simulink model "Nonlinear_Performance_Simulation_NAPE_ANTONIO_CAROTENUTO"  (R2023b)
settings: Solver=ode45  StartTime=0.0  StopTime=305.0  RelTol=1e-3  AbsTol=1e-6
undefined symbols (not defined in the file or in its folder): alpha0L, altitude_0, bankAngle_0, bankAngleMax, flightPathAngle_0, flightPathAngle_c1, flightPathAngle_c2, flightPathAngle_c3, flightPathAngle_c4, headingAngle_0, headingAngle_c1, headingAngle_c2, headingAngle_c3, headingAngle_c4, kD0, kD1, kL, kLI, kLP, kNu, kTI, kTP, kWdot, lift_0, mass_0, pL, pNu, pT, speed_0, speed_c1, speed_c2, speed_c3, speed_c4, thrust_0, thrustMax, wind_0, xE_0, yE_0
libraries: aerolibatmos2 x1
settings Model: Creator=agodemar  LastModifiedBy=sasi
settings SolverCC: AutoScaleAbsTol=off  AlgebraicLoopSolver=TrustRegion
settings DataIOCC: SaveFormat=Array  SignalLoggingSaveFormat=ModelDataLogs  ReturnWorkspaceOutputs=off
settings OptimizationCC: BlockReduction=off  BooleanDataType=off  LifeSpan=inf
settings DebuggingCC: SaveWithParameterizedLinksMsg=none  UnderspecifiedInitializationDetection=Classic  MergeDetectMultiDrivingBlocksExec=none  SignalResolutionControl=TryResolveAllWithWarning  MultiTaskDSMMsg=warning  MultiTaskCondExecSysMsg=none  UnconnectedInputMsg=warning  UnconnectedOutputMsg=warning  UnconnectedLineMsg=warning  SFUnexpectedBacktrackingDiag=warning  SFNoUnconditionalDefaultTransitionDiag=warning  ArithmeticOperatorsInVariantConditions=warning
settings HardwareCC: TargetUnknown=on
settings ModelReferenceCC: EnableRefExpFcnMdlSchedulingChecks=on  PropagateSignalLabelsOutOfModel=off
settings SFSimCC: SimUseLocalCustomCode=off  CustomCodeUndefinedFunction=UseInterfaceOnly
settings RTWCC: RTWUseLocalCustomCode=off
settings CodeAppCC: StateflowObjectComments=on
settings GRTTargetCC: TargetLangStandard=C89/C90 (ANSI)  CombineOutputUpdateFcns=off  GRTInterface=on
settings ConfigComp: CovMetricSettings=dw  CovSaveCumulativeToWorkspaceVar=on  CovSaveSingleToWorkspaceVar=on  CovExternalEMLEnable=off

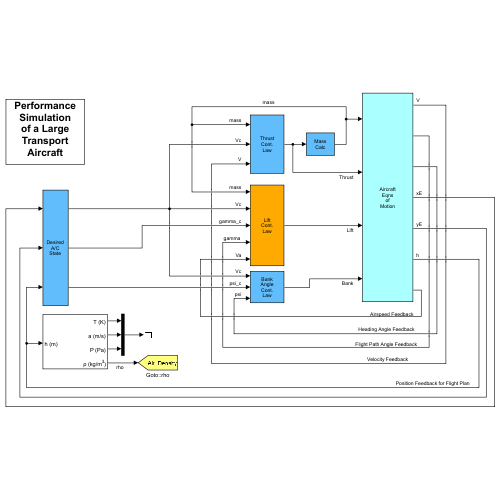
[thumbnail: Simulink's stored preview of the top-level diagram]
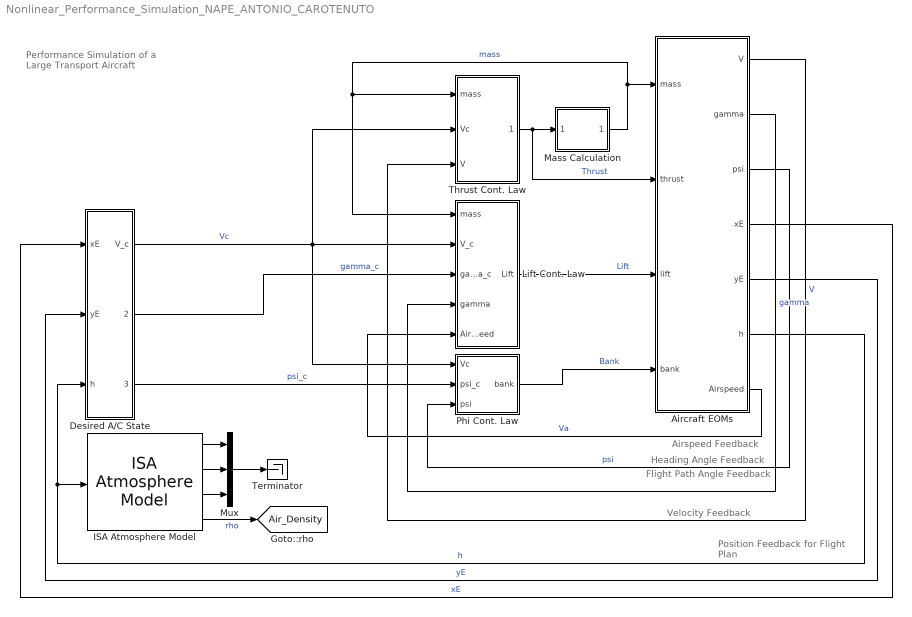
== system Nonlinear_Performance_Simulation_NAPE_ANTONIO_CAROTENUTO ==
  note: Performance Simulation
      | of a Large Transport Aircraft
  note: Velocity Feedback
  note: Flight Path Angle Feedback
  note: Heading Angle Feedback
  note: Position Feedback for Flight Plan
  note: Airspeed Feedback
  Aircraft EOMs : Subsystem
      mask Display: disp('Aircraft\nEqns\nof\nMotion')
  Desired A/C State : Subsystem
      mask Display: disp('Desired\nA/C\nState')
  ISA Atmosphere Model : aerolibatmos2/ISA Atmosphere Model  useExtended=off  action=Warning  custom=off  viscosityOut=off  g=9.80665  gamma=1.4  R=287.0531  L=0.0065  h_trop=11000  h_strat=20000  rho0=1.225  P0=101325  T0=288.15  h0=0
  Lift Cont. Law : Subsystem
      mask Display: disp('Lift\nCont.\nLaw')
  Mass Calculation : Subsystem
      mask Display: disp('Mass\nCalc')
  Mux : Mux  Inputs=3
  Phi Cont. Law : Subsystem
      mask Display: disp('Bank\nAngle\nCont.\nLaw')
  Terminator : Terminator
  Thrust Cont. Law : Subsystem
      mask Display: disp('Thrust\nCont.\nLaw')
  tag scope: Air_Density=global
  wires:
  Phi Cont. Law/1(bank) -> Aircraft EOMs/4(bank)  "Bank"
  Mass Calculation/1("Mass ") -> Lift Cont. Law/1(mass), Thrust Cont. Law/1(mass), Aircraft EOMs/1("mass ")  "mass"
  Lift Cont. Law/1(Lift) -> Aircraft EOMs/3("lift ")  "Lift"
  Thrust Cont. Law/1(Thrust) -> Aircraft EOMs/2("thrust "), Mass Calculation/1(thrust)  "Thrust"
  Desired A/C State/1(V_c) -> Phi Cont. Law/1(Vc), Thrust Cont. Law/2(Vc), Lift Cont. Law/2(V_c)  "Vc"
  Desired A/C State/2(gamma_c) -> Lift Cont. Law/3(gamma_c)  "gamma_c"
  Desired A/C State/3(psi_c) -> Phi Cont. Law/2(psi_c)  "psi_c"
  Aircraft EOMs/3(" psi ") -> Phi Cont. Law/3(psi)  "psi"
  Aircraft EOMs/2(" gamma ") -> Lift Cont. Law/4(gamma)  "gamma"
  Aircraft EOMs/1(" V ") -> Thrust Cont. Law/3(V)  "V"
  Aircraft EOMs/7(Airspeed) -> Lift Cont. Law/5(Airspeed)  "Va"
  Aircraft EOMs/6(h) -> Desired A/C State/3(h), ISA Atmosphere Model/1  "h"
  Aircraft EOMs/5(yE) -> Desired A/C State/2(yE)  "yE"
  Aircraft EOMs/4(xE) -> Desired A/C State/1(xE)  "xE"
  Mux/1 -> Terminator/1
  ISA Atmosphere Model/1 -> Mux/1
  ISA Atmosphere Model/2 -> Mux/2
  ISA Atmosphere Model/3 -> Mux/3
  ISA Atmosphere Model/4 -> [Air_Density]  "rho"

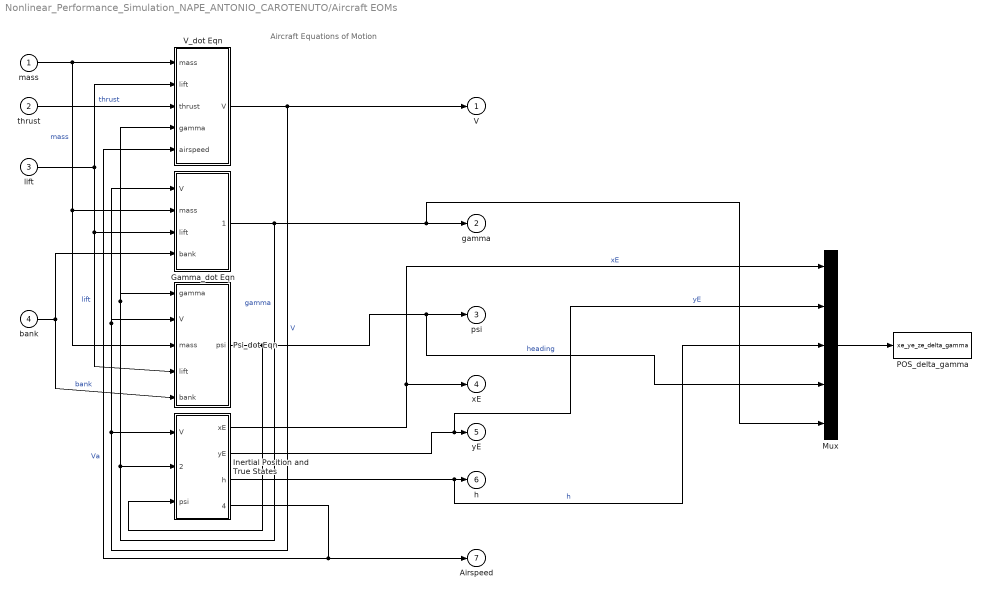
== system Nonlinear_Performance_Simulation_NAPE_ANTONIO_CAROTENUTO/Aircraft EOMs ==
  note: Aircraft Equations of Motion
  "mass " : Inport
  "thrust " : Inport  Port=2
  "lift " : Inport  Port=3
  bank : Inport  Port=4
  Gamma_dot Eqn : Subsystem
      mask Display: disp('Gam_dot\nEqn')
  Inertial Position and True States : Subsystem
      mask Display: disp('Inertial\nPosition\nand\nAirspeed')
  Mux : Mux  Inputs=5
  POS_delta_gamma : ToWorkspace  VariableName=xe_ye_ze_delta_gamma  SaveFormat=Timeseries  SampleTime=-1
  Psi_dot Eqn : Subsystem
      mask Display: disp('Psi_dot\nEqn')
  V_dot Eqn : Subsystem
      mask Display: disp('V_dot\nEqn')
  " V " : Outport
  " gamma " : Outport  Port=2
  " psi " : Outport  Port=3
  xE : Outport  Port=4
  yE : Outport  Port=5
  h : Outport  Port=6
  Airspeed : Outport  Port=7
  wires:
  bank/1 -> Psi_dot Eqn/5(bank), Gamma_dot Eqn/4(bank)  "bank"
  "lift "/1 -> V_dot Eqn/2(lift), Psi_dot Eqn/4("lift "), Gamma_dot Eqn/3("lift ")  "lift"
  "mass "/1 -> Psi_dot Eqn/3(mass), Gamma_dot Eqn/2(mass), V_dot Eqn/1(mass)  "mass"
  "thrust "/1 -> V_dot Eqn/3(thrust)  "thrust"
  Psi_dot Eqn/1(psi) -> Mux/4, " psi "/1, Inertial Position and True States/3(psi)  "heading"
  Gamma_dot Eqn/1(Gamma) -> Mux/5, " gamma "/1, V_dot Eqn/4(gamma), Psi_dot Eqn/1(gamma), Inertial Position and True States/2("gamma ")  "gamma"
  V_dot Eqn/1(V) -> Gamma_dot Eqn/1(V), Psi_dot Eqn/2(V), Inertial Position and True States/1(V), " V "/1  "V"
  Inertial Position and True States/2(yE) -> Mux/2, yE/1  "yE"
  Inertial Position and True States/3(h) -> Mux/3, h/1  "h"
  Inertial Position and True States/1(xE) -> Mux/1, xE/1  "xE"
  Inertial Position and True States/4(AirSpeed) -> V_dot Eqn/5(airspeed), Airspeed/1  "Va"
  Mux/1 -> POS_delta_gamma/1

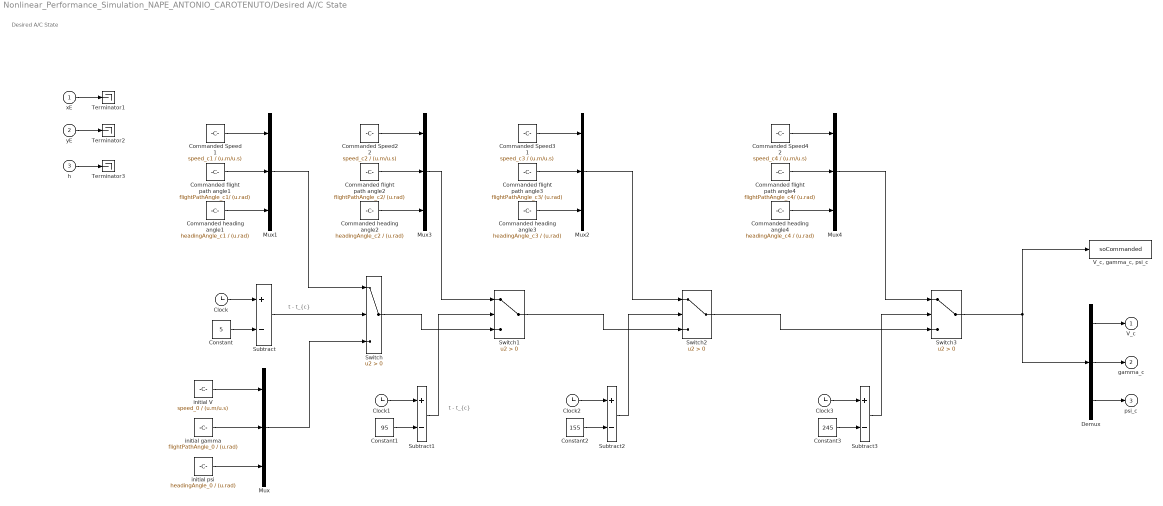
== system Nonlinear_Performance_Simulation_NAPE_ANTONIO_CAROTENUTO/Desired A//C State ==
  note: t - t_{c}
  note: Desired A/C State
  note: t - t_{c}
  xE : Inport
  yE : Inport  Port=2
  h : Inport  Port=3
  Clock{,1..3} (4 alike) : Clock
  Commanded Speed 1 : Constant  Value=speed_c1 / (u.m/u.s)
  Commanded Speed2 2 : Constant  Value=speed_c2 / (u.m/u.s)
  Commanded Speed3 1 : Constant  Value=speed_c3 / (u.m/u.s)
  Commanded Speed4 2 : Constant  Value=speed_c4 / (u.m/u.s)
  Commanded flight path angle1 : Constant  Value=flightPathAngle_c1/ (u.rad)
  Commanded flight path angle2 : Constant  Value=flightPathAngle_c2/ (u.rad)
  Commanded flight path angle3 : Constant  Value=flightPathAngle_c3/ (u.rad)
  Commanded flight path angle4 : Constant  Value=flightPathAngle_c4/ (u.rad)
  Commanded heading angle1 : Constant  Value=headingAngle_c1 / (u.rad)
  Commanded heading angle2 : Constant  Value=headingAngle_c2 / (u.rad)
  Commanded heading angle3 : Constant  Value=headingAngle_c3 / (u.rad)
  Commanded heading angle4 : Constant  Value=headingAngle_c4 / (u.rad)
  Constant : Constant  Value=5
  Constant1 : Constant  Value=95
  Constant2 : Constant  Value=155
  Constant3 : Constant  Value=245
  Demux : Demux  Outputs=3
  Mux{,1..4} (5 alike) : Mux  Inputs=3
  Subtract{,1..3} (4 alike) : Sum  Inputs=+-
  Switch{,1..3} (4 alike) : Switch  Criteria=u2 > Threshold  SaturateOnIntegerOverflow=off  InputSameDT=off
  Terminator1 : Terminator
  Terminator2 : Terminator
  Terminator3 : Terminator
  "V_c, gamma_c, psi_c" : ToWorkspace  VariableName=soCommanded  SaveFormat=Timeseries  SampleTime=-1
  initial V : Constant  Value=speed_0 / (u.m/u.s)
  initial gamma : Constant  Value=flightPathAngle_0 / (u.rad)
  initial psi : Constant  Value=headingAngle_0 / (u.rad)
  V_c : Outport
  gamma_c : Outport  Port=2
  psi_c : Outport  Port=3
  wires:
  xE/1 -> Terminator1/1
  yE/1 -> Terminator2/1
  h/1 -> Terminator3/1
  Constant/1 -> Subtract/2
  Clock/1 -> Subtract/1
  initial gamma/1 -> Mux/2
  initial V/1 -> Mux/1
  initial psi/1 -> Mux/3
  Mux/1 -> Switch/3
  Subtract/1 -> Switch/2
  Demux/1 -> V_c/1
  Demux/2 -> gamma_c/1
  Demux/3 -> psi_c/1
  Switch/1 -> Switch1/3
  Commanded flight path angle2/1 -> Mux3/2
  Commanded heading angle2/1 -> Mux3/3
  Commanded Speed2 2/1 -> Mux3/1
  Mux1/1 -> Switch/1
  Commanded Speed 1/1 -> Mux1/1
  Commanded flight path angle1/1 -> Mux1/2
  Commanded heading angle1/1 -> Mux1/3
  Mux3/1 -> Switch1/1
  Subtract1/1 -> Switch1/2
  Constant1/1 -> Subtract1/2
  Clock1/1 -> Subtract1/1
  Commanded flight path angle3/1 -> Mux2/2
  Commanded heading angle3/1 -> Mux2/3
  Mux2/1 -> Switch2/1
  Commanded Speed3 1/1 -> Mux2/1
  Switch1/1 -> Switch2/3
  Constant2/1 -> Subtract2/2
  Clock2/1 -> Subtract2/1
  Subtract2/1 -> Switch2/2
  Commanded Speed4 2/1 -> Mux4/1
  Commanded flight path angle4/1 -> Mux4/2
  Switch2/1 -> Switch3/3
  Clock3/1 -> Subtract3/1
  Commanded heading angle4/1 -> Mux4/3
  Constant3/1 -> Subtract3/2
  Subtract3/1 -> Switch3/2
  Mux4/1 -> Switch3/1
  Switch3/1 -> "V_c, gamma_c, psi_c"/1, Demux/1

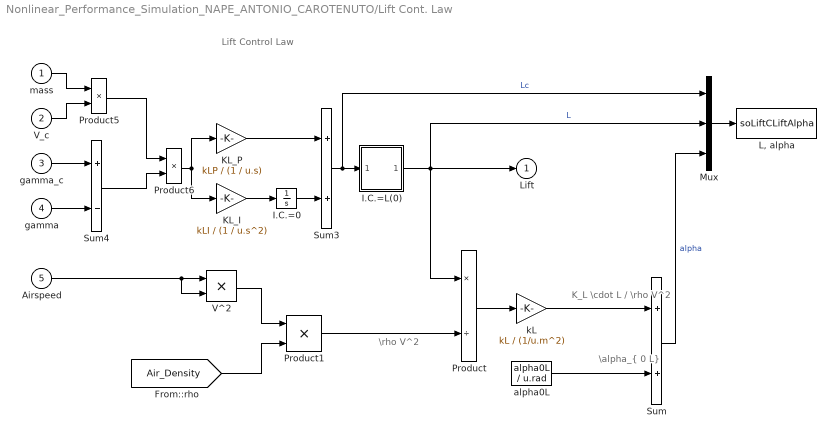
== system Nonlinear_Performance_Simulation_NAPE_ANTONIO_CAROTENUTO/Lift Cont. Law ==
  note: \rho V^2
  note: Lift Control Law
  note: K_L \cdot L / \rho V^2
  note: \alpha_{ 0 L}
  mass : Inport
  V_c : Inport  Port=2
  gamma_c : Inport  Port=3
  gamma : Inport  Port=4
  Airspeed : Inport  Port=5
  I.C.=0 : Integrator  InitialCondition=lift_0 / (u.N)
  I.C.=L(0) : Subsystem
      mask Display: disp('pL\n-----\ns + pL')
  KL_I : Gain  Gain=kLI / (1 / u.s^2)  SaturateOnIntegerOverflow=on  OutDataTypeStr=Inherit: Same as input  ParamDataTypeStr=Inherit: Same as input
  KL_P : Gain  Gain=kLP / (1 / u.s)  SaturateOnIntegerOverflow=on  OutDataTypeStr=Inherit: Same as input  ParamDataTypeStr=Inherit: Same as input
  "L, alpha" : ToWorkspace  VariableName=soLiftCLiftAlpha  SaveFormat=Timeseries  SampleTime=-1
  Mux : Mux  Inputs=3
  Product : Product  Inputs=*/
  Product1 : Product  InputSameDT=on  RndMeth=Zero  SaturateOnIntegerOverflow=on  OutDataTypeStr=Inherit: Same as first input
  Product5 : Product  InputSameDT=on  RndMeth=Zero  SaturateOnIntegerOverflow=on  OutDataTypeStr=Inherit: Same as first input
  Product6 : Product  InputSameDT=on  RndMeth=Zero  SaturateOnIntegerOverflow=on  OutDataTypeStr=Inherit: Same as first input
  Sum : Sum  InputSameDT=on  SaturateOnIntegerOverflow=on  OutDataTypeStr=Inherit: Same as first input
  Sum3 : Sum  InputSameDT=on  SaturateOnIntegerOverflow=on  OutDataTypeStr=Inherit: Same as first input
  Sum4 : Sum  Inputs=+-  InputSameDT=on  SaturateOnIntegerOverflow=on  OutDataTypeStr=Inherit: Same as first input
  V^2 : Product  InputSameDT=on  RndMeth=Zero  SaturateOnIntegerOverflow=on  OutDataTypeStr=Inherit: Same as first input
  alpha0L : Constant  Value=alpha0L / u.rad
  kL : Gain  Gain=kL / (1/u.m^2)  SaturateOnIntegerOverflow=on  OutDataTypeStr=Inherit: Same as input  ParamDataTypeStr=Inherit: Same as input
  Lift : Outport
  wires:
  I.C.=L(0)/1(Out1 L(t)) -> Mux/2, Product/1, Lift/1  "L"
  Sum3/1 -> Mux/1, I.C.=L(0)/1(In1 Lc(t))  "Lc"
  gamma/1 -> Sum4/2
  gamma_c/1 -> Sum4/1
  Sum4/1 -> Product6/2
  V_c/1 -> Product5/2
  mass/1 -> Product5/1
  Product5/1 -> Product6/1
  Product6/1 -> KL_I/1, KL_P/1
  KL_P/1 -> Sum3/1
  I.C.=0/1 -> Sum3/2
  KL_I/1 -> I.C.=0/1
  Airspeed/1 -> V^2/1, V^2/2
  Product/1 -> kL/1
  kL/1 -> Sum/1
  Sum/1 -> Mux/3  "alpha"
  alpha0L/1 -> Sum/2
  V^2/1 -> Product1/1
  [Air_Density] -> Product1/2
  Product1/1 -> Product/2
  Mux/1 -> "L, alpha"/1

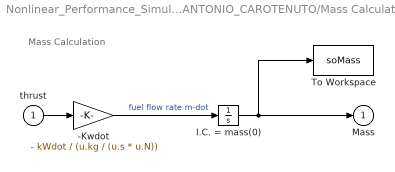
== system Nonlinear_Performance_Simulation_NAPE_ANTONIO_CAROTENUTO/Mass Calculation ==
  note: Mass Calculation
  thrust : Inport
  -Kwdot : Gain  Gain=- kWdot / (u.kg / (u.s * u.N))  SaturateOnIntegerOverflow=on  OutDataTypeStr=Inherit: Same as input  ParamDataTypeStr=Inherit: Same as input
  I.C. = mass(0) : Integrator  InitialCondition=mass_0 / u.kg
  To Workspace : ToWorkspace  VariableName=soMass  SaveFormat=Timeseries  SampleTime=-1
  "Mass " : Outport
  wires:
  -Kwdot/1 -> I.C. = mass(0)/1  "fuel flow rate m-dot"
  I.C. = mass(0)/1 -> To Workspace/1, "Mass "/1
  thrust/1 -> -Kwdot/1

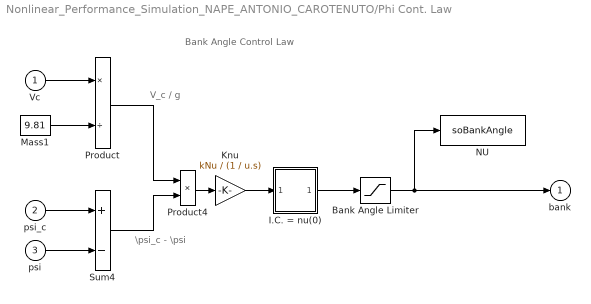
== system Nonlinear_Performance_Simulation_NAPE_ANTONIO_CAROTENUTO/Phi Cont. Law ==
  note: V_c / g
  note: Bank Angle Control Law
  note: \psi_c - \psi
  Vc : Inport
  psi_c : Inport  Port=2
  psi : Inport  Port=3
  Bank Angle Limiter : Saturate  UpperLimit=bankAngleMax / u.rad  LowerLimit=- bankAngleMax / u.rad
  I.C. = nu(0) : Subsystem
      mask Display: disp('pf\n-----\ns + pf')
  Knu : Gain  Gain=kNu / (1 / u.s)  SaturateOnIntegerOverflow=on  OutDataTypeStr=Inherit: Same as input  ParamDataTypeStr=Inherit: Same as input
  Mass1 : Constant  Value=9.81
  NU : ToWorkspace  VariableName=soBankAngle  SaveFormat=Timeseries  SampleTime=-1
  Product : Product  Inputs=*/
  Product4 : Product  InputSameDT=on  RndMeth=Zero  SaturateOnIntegerOverflow=on  OutDataTypeStr=Inherit: Same as first input
  Sum4 : Sum  Inputs=+-  InputSameDT=on  SaturateOnIntegerOverflow=on  OutDataTypeStr=Inherit: Same as first input
  bank : Outport
  wires:
  I.C. = nu(0)/1(Out1 nu) -> Bank Angle Limiter/1
  Knu/1 -> I.C. = nu(0)/1(In1 nu_c)
  Product4/1 -> Knu/1
  psi/1 -> Sum4/2
  psi_c/1 -> Sum4/1
  Sum4/1 -> Product4/2
  Vc/1 -> Product/1
  Mass1/1 -> Product/2
  Bank Angle Limiter/1 -> NU/1, bank/1
  Product/1 -> Product4/1

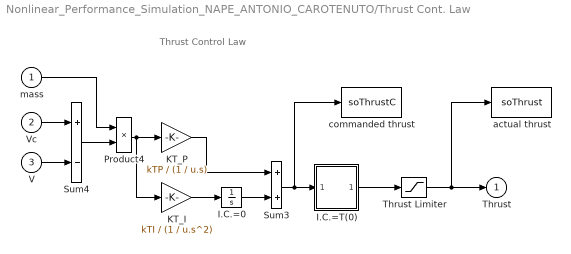
== system Nonlinear_Performance_Simulation_NAPE_ANTONIO_CAROTENUTO/Thrust Cont. Law ==
  note: Thrust Control Law
  mass : Inport
  Vc : Inport  Port=2
  V : Inport  Port=3
  I.C.=0 : Integrator  InitialCondition=thrust_0 / u.N
  I.C.=T(0) : Subsystem
      mask Display: disp('pT\n-----\ns + pT')
  KT_I : Gain  Gain=kTI / (1 / u.s^2)  SaturateOnIntegerOverflow=on  OutDataTypeStr=Inherit: Same as input  ParamDataTypeStr=Inherit: Same as input
  KT_P : Gain  Gain=kTP / (1 / u.s)  SaturateOnIntegerOverflow=on  OutDataTypeStr=Inherit: Same as input  ParamDataTypeStr=Inherit: Same as input
  Product4 : Product  InputSameDT=on  RndMeth=Zero  SaturateOnIntegerOverflow=on  OutDataTypeStr=Inherit: Same as first input
  Sum3 : Sum  InputSameDT=on  SaturateOnIntegerOverflow=on  OutDataTypeStr=Inherit: Same as first input
  Sum4 : Sum  Inputs=+-  InputSameDT=on  SaturateOnIntegerOverflow=on  OutDataTypeStr=Inherit: Same as first input
  Thrust Limiter : Saturate  UpperLimit=thrustMax / u.N  LowerLimit=0
  actual thrust : ToWorkspace  VariableName=soThrust  SaveFormat=Timeseries  SampleTime=-1
  commanded thrust : ToWorkspace  VariableName=soThrustC  SaveFormat=Timeseries  SampleTime=-1
  Thrust : Outport
  wires:
  Thrust Limiter/1 -> actual thrust/1, Thrust/1
  I.C.=T(0)/1(Out1 T(t)) -> Thrust Limiter/1
  Sum3/1 -> commanded thrust/1, I.C.=T(0)/1(In1 Tc(t))
  Product4/1 -> KT_I/1, KT_P/1
  V/1 -> Sum4/2
  Vc/1 -> Sum4/1
  mass/1 -> Product4/1
  Sum4/1 -> Product4/2
  KT_P/1 -> Sum3/1
  I.C.=0/1 -> Sum3/2
  KT_I/1 -> I.C.=0/1

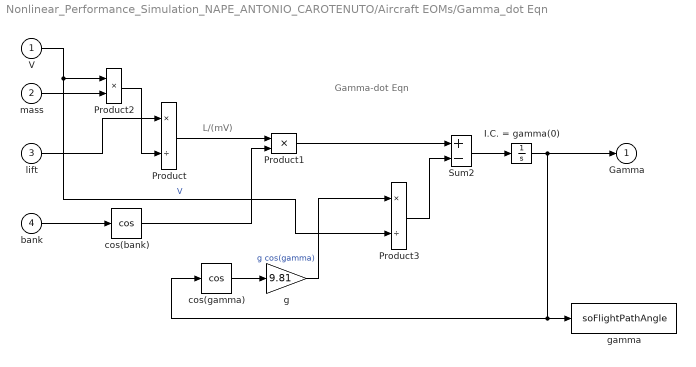
== system Nonlinear_Performance_Simulation_NAPE_ANTONIO_CAROTENUTO/Aircraft EOMs/Gamma_dot Eqn ==
  note: L/(mV)
  note: Gamma-dot Eqn
  V : Inport
  mass : Inport  Port=2
  "lift " : Inport  Port=3
  bank : Inport  Port=4
  I.C. = gamma(0) : Integrator  InitialCondition=flightPathAngle_0 / u.rad
  Product : Product  Inputs=*/
  Product1 : Product  InputSameDT=on  RndMeth=Zero  SaturateOnIntegerOverflow=on  OutDataTypeStr=Inherit: Same as first input
  Product2 : Product  InputSameDT=on  RndMeth=Zero  SaturateOnIntegerOverflow=on  OutDataTypeStr=Inherit: Same as first input
  Product3 : Product  Inputs=*/
  Sum2 : Sum  Inputs=+-  InputSameDT=on  SaturateOnIntegerOverflow=on  OutDataTypeStr=Inherit: Same as first input
  cos(bank) : Trigonometry  Operator=cos
  cos(gamma) : Trigonometry  Operator=cos
  g : Gain  Gain=9.81
  gamma : ToWorkspace  VariableName=soFlightPathAngle  SaveFormat=Timeseries  SampleTime=-1
  Gamma : Outport
  wires:
  cos(bank)/1 -> Product1/2
  bank/1 -> cos(bank)/1
  "lift "/1 -> Product/1
  I.C. = gamma(0)/1 -> Gamma/1, gamma/1, cos(gamma)/1
  mass/1 -> Product2/2
  V/1 -> Product3/2, Product2/1  "V"
  Sum2/1 -> I.C. = gamma(0)/1
  g/1 -> Product3/1  "g cos(gamma)"
  cos(gamma)/1 -> g/1
  Product1/1 -> Sum2/1
  Product/1 -> Product1/1
  Product2/1 -> Product/2
  Product3/1 -> Sum2/2

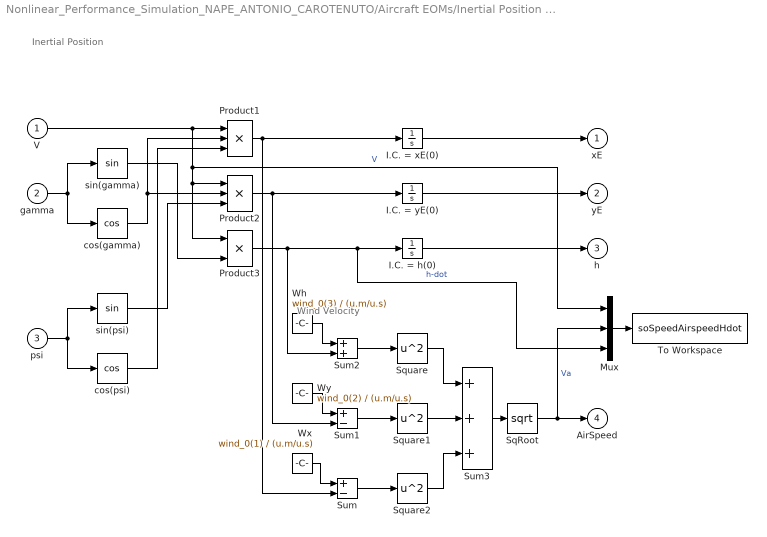
== system Nonlinear_Performance_Simulation_NAPE_ANTONIO_CAROTENUTO/Aircraft EOMs/Inertial Position and True States ==
  note: Wind Velocity
  note: Inertial Position
  V : Inport
  "gamma " : Inport  Port=2
  psi : Inport  Port=3
  I.C. = h(0) : Integrator  InitialCondition=altitude_0 / u.m
  I.C. = xE(0) : Integrator  InitialCondition=xE_0 / u.m
  I.C. = yE(0) : Integrator  InitialCondition=yE_0 / u.m
  Mux : Mux  Inputs=3
  Product1 : Product  Inputs=3  InputSameDT=on  RndMeth=Zero  SaturateOnIntegerOverflow=on  OutDataTypeStr=Inherit: Same as first input
  Product2 : Product  Inputs=3  InputSameDT=on  RndMeth=Zero  SaturateOnIntegerOverflow=on  OutDataTypeStr=Inherit: Same as first input
  Product3 : Product  InputSameDT=on  RndMeth=Zero  SaturateOnIntegerOverflow=on  OutDataTypeStr=Inherit: Same as first input
  SqRoot : Math  Operator=sqrt  SignedPower=on
  Square : Math  Operator=square  SignedPower=on
  Square1 : Math  Operator=square  SignedPower=on
  Square2 : Math  Operator=square  SignedPower=on
  Sum : Sum  Inputs=+-  InputSameDT=on  SaturateOnIntegerOverflow=on  OutDataTypeStr=Inherit: Same as first input
  Sum1 : Sum  Inputs=+-  InputSameDT=on  SaturateOnIntegerOverflow=on  OutDataTypeStr=Inherit: Same as first input
  Sum2 : Sum  InputSameDT=on  SaturateOnIntegerOverflow=on  OutDataTypeStr=Inherit: Same as first input
  Sum3 : Sum  Inputs=+++  InputSameDT=on  SaturateOnIntegerOverflow=on  OutDataTypeStr=Inherit: Same as first input
  To Workspace : ToWorkspace  VariableName=soSpeedAirspeedHdot  SaveFormat=Timeseries  SampleTime=-1
  Wh : Constant  Value=wind_0(3) / (u.m/u.s)
  Wx : Constant  Value=wind_0(1) / (u.m/u.s)
  Wy : Constant  Value=wind_0(2) / (u.m/u.s)
  cos(gamma) : Trigonometry  Operator=cos
  cos(psi) : Trigonometry  Operator=cos
  sin(gamma) : Trigonometry
  sin(psi) : Trigonometry
  xE : Outport
  yE : Outport  Port=2
  h : Outport  Port=3
  AirSpeed : Outport  Port=4
  wires:
  "gamma "/1 -> cos(gamma)/1, sin(gamma)/1
  psi/1 -> sin(psi)/1, cos(psi)/1
  cos(psi)/1 -> Product1/3
  V/1 -> Mux/1, Product2/1, Product3/1, Product1/1  "V"
  cos(gamma)/1 -> Product1/2, Product2/2
  sin(psi)/1 -> Product2/3
  sin(gamma)/1 -> Product3/2
  I.C. = xE(0)/1 -> xE/1
  I.C. = yE(0)/1 -> yE/1
  I.C. = h(0)/1 -> h/1
  Product3/1 -> Mux/3, I.C. = h(0)/1, Sum2/2  "h-dot"
  Product2/1 -> I.C. = yE(0)/1, Sum1/2
  Product1/1 -> I.C. = xE(0)/1, Sum/2
  Wx/1 -> Sum/1
  Wy/1 -> Sum1/1
  Wh/1 -> Sum2/1
  Sum2/1 -> Square/1
  Sum1/1 -> Square1/1
  Sum/1 -> Square2/1
  Sum3/1 -> SqRoot/1
  SqRoot/1 -> Mux/2, AirSpeed/1  "Va"
  Square1/1 -> Sum3/2
  Square/1 -> Sum3/1
  Square2/1 -> Sum3/3
  Mux/1 -> To Workspace/1

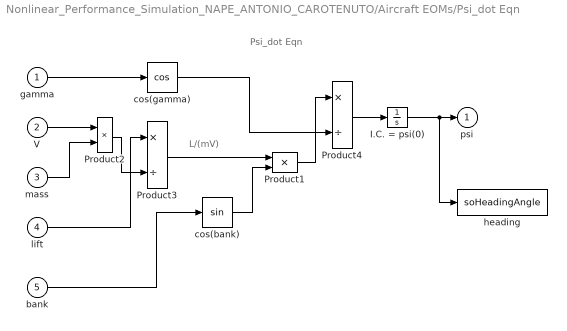
== system Nonlinear_Performance_Simulation_NAPE_ANTONIO_CAROTENUTO/Aircraft EOMs/Psi_dot Eqn ==
  note: Psi_dot Eqn
  note: L/(mV)
  gamma : Inport
  V : Inport  Port=2
  mass : Inport  Port=3
  "lift " : Inport  Port=4
  bank : Inport  Port=5
  I.C. = psi(0) : Integrator  InitialCondition=headingAngle_0 / u.rad
  Product1 : Product  InputSameDT=on  RndMeth=Zero  SaturateOnIntegerOverflow=on  OutDataTypeStr=Inherit: Same as first input
  Product2 : Product  InputSameDT=on  RndMeth=Zero  SaturateOnIntegerOverflow=on  OutDataTypeStr=Inherit: Same as first input
  Product3 : Product  Inputs=*/  InputSameDT=on  RndMeth=Zero  SaturateOnIntegerOverflow=on  OutDataTypeStr=Inherit: Same as first input
  Product4 : Product  Inputs=*/  InputSameDT=on  RndMeth=Zero  SaturateOnIntegerOverflow=on  OutDataTypeStr=Inherit: Same as first input
  cos(bank) : Trigonometry
  cos(gamma) : Trigonometry  Operator=cos
  heading : ToWorkspace  VariableName=soHeadingAngle  SaveFormat=Timeseries  SampleTime=-1
  psi : Outport
  wires:
  Product4/1 -> I.C. = psi(0)/1
  cos(gamma)/1 -> Product4/2
  Product1/1 -> Product4/1
  gamma/1 -> cos(gamma)/1
  cos(bank)/1 -> Product1/2
  bank/1 -> cos(bank)/1
  I.C. = psi(0)/1 -> heading/1, psi/1
  mass/1 -> Product2/2
  V/1 -> Product2/1
  Product3/1 -> Product1/1
  "lift "/1 -> Product3/1
  Product2/1 -> Product3/2

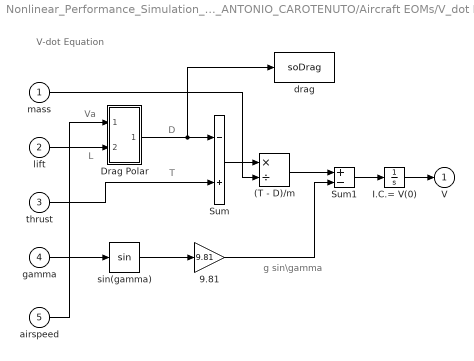
== system Nonlinear_Performance_Simulation_NAPE_ANTONIO_CAROTENUTO/Aircraft EOMs/V_dot Eqn ==
  note: g sin\gamma
  note: V-dot Equation
  note: T
  note: D
  note: Va
  note: L
  mass : Inport
  lift : Inport  Port=2
  thrust : Inport  Port=3
  gamma : Inport  Port=4
  airspeed : Inport  Port=5
  (T - D)/m : Product  Inputs=*/
  9.81 : Gain  Gain=9.81
  Drag Polar : Subsystem
      mask Display: disp('Drag\nPolar')
  I.C.= V(0) : Integrator  InitialCondition=speed_0 / (u.m/u.s)
  Sum : Sum  Inputs=-+  InputSameDT=on  SaturateOnIntegerOverflow=on  OutDataTypeStr=Inherit: Same as first input
  Sum1 : Sum  Inputs=+-  InputSameDT=on  SaturateOnIntegerOverflow=on  OutDataTypeStr=Inherit: Same as first input
  drag : ToWorkspace  VariableName=soDrag  SaveFormat=Timeseries  SampleTime=-1
  sin(gamma) : Trigonometry
  V : Outport
  wires:
  gamma/1 -> sin(gamma)/1
  lift/1 -> Drag Polar/2(Lift)
  sin(gamma)/1 -> 9.81/1
  (T - D)/m/1 -> Sum1/1
  9.81/1 -> Sum1/2
  Sum1/1 -> I.C.= V(0)/1
  I.C.= V(0)/1 -> V/1
  airspeed/1 -> Drag Polar/1(Airspeed)
  thrust/1 -> Sum/2
  Drag Polar/1(Drag) -> drag/1, Sum/1
  mass/1 -> (T - D)/m/2
  Sum/1 -> (T - D)/m/1

== system Nonlinear_Performance_Simulation_NAPE_ANTONIO_CAROTENUTO/Lift Cont. Law/I.C.=L(0) ==
  note: x = L(t), u = L_c(t)
  In1 Lc(t) : Inport
  I.C.=L(0) : StateSpace  A=- pL / (1/u.s)  B=pL / (1/u.s)  D=0  InitialCondition=lift_0 / u.N
  Out1 L(t) : Outport
  wires:
  In1 Lc(t)/1 -> I.C.=L(0)/1
  I.C.=L(0)/1 -> Out1 L(t)/1

== system Nonlinear_Performance_Simulation_NAPE_ANTONIO_CAROTENUTO/Phi Cont. Law/I.C. = nu(0) ==
  note: A = -pNu, B = pNu
  note: x(t) = nu(t), u(t) = nu_c(t)
  In1 nu_c : Inport
  I.C. = nu(0) : StateSpace  A=-pNu / (1 / u.s)  B=pNu / (1 / u.s)  D=0  InitialCondition=bankAngle_0 / u.rad
  Out1 nu : Outport
  wires:
  In1 nu_c/1 -> I.C. = nu(0)/1
  I.C. = nu(0)/1 -> Out1 nu/1

== system Nonlinear_Performance_Simulation_NAPE_ANTONIO_CAROTENUTO/Thrust Cont. Law/I.C.=T(0) ==
  note: x = T(t), u = T_c(t)
  In1 Tc(t) : Inport
  I.C.=T(0) : StateSpace  A=-pT / (u.rad/u.s)  B=pT / (u.rad/u.s)  D=0  InitialCondition=thrust_0 / (u.N)
  Out1 T(t) : Outport
  wires:
  In1 Tc(t)/1 -> I.C.=T(0)/1
  I.C.=T(0)/1 -> Out1 T(t)/1

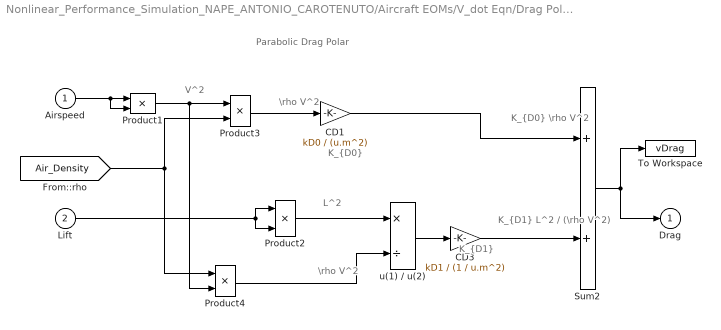
== system Nonlinear_Performance_Simulation_NAPE_ANTONIO_CAROTENUTO/Aircraft EOMs/V_dot Eqn/Drag Polar ==
  note: Parabolic Drag Polar
  note: V^2
  note: L^2
  note: K_{D0} \rho V^2
  note: K_{D0}
  note: K_{D1}
  note: \rho V^2
  note: \rho V^2
  note: K_{D1} L^2 / (\rho V^2)
  Airspeed : Inport
  Lift : Inport  Port=2
  CD1 : Gain  Gain=kD0 / (u.m^2)  SaturateOnIntegerOverflow=on  OutDataTypeStr=Inherit: Same as input  ParamDataTypeStr=Inherit: Same as input
  CD3 : Gain  Gain=kD1 / (1 / u.m^2)  SaturateOnIntegerOverflow=on  OutDataTypeStr=Inherit: Same as input  ParamDataTypeStr=Inherit: Same as input
  Product{1..4} (4 alike) : Product  InputSameDT=on  RndMeth=Zero  SaturateOnIntegerOverflow=on  OutDataTypeStr=Inherit: Same as first input
  Sum2 : Sum  InputSameDT=on  SaturateOnIntegerOverflow=on  OutDataTypeStr=Inherit: Same as first input
  To Workspace : ToWorkspace  VariableName=vDrag
  u(1) / u(2) : Product  Inputs=*/
  Drag : Outport
  wires:
  Lift/1 -> Product2/1, Product2/2
  Airspeed/1 -> Product1/2, Product1/1
  Product1/1 -> Product4/2, Product3/1
  Sum2/1 -> To Workspace/1, Drag/1
  [Air_Density] -> Product3/2, Product4/1
  Product2/1 -> u(1) / u(2)/1
  u(1) / u(2)/1 -> CD3/1
  Product4/1 -> u(1) / u(2)/2
  Product3/1 -> CD1/1
  CD1/1 -> Sum2/1
  CD3/1 -> Sum2/2
